simulink model "MIL4L3_SW6_V1_20220211"  (R2018b)
settings: Solver=FixedStepAuto  StartTime=0.0  StopTime=inf  FixedStep=0.001  RelTol=1e-3
PreLoadFcn:
  | A0_MILtest;
undefined symbols (not defined in the file or in its folder): Clb_ICADirect_LaneDisp_StateFive, Clb_ICADirect_LaneDisp_StateFour, Clb_ICADirect_LaneDisp_StateOne, Clb_ICADirect_LaneDisp_StateThree, Clb_ICADirect_LaneDisp_StateTwo, Clb_ICADirect_LaneDisp_StateZero, Clb_ICADirect_LaneDispSW, Clb_ICADirect_TrnLghtsCom_Switch, Clb_ICADirect_TrnLghtsCom_Value, Clb_ICADirect_TrnLghtsCrtl_Inhb, IMAP_Clb_ACU_Driver_Belt, IMAP_Clb_ACU_Driver_Belt_Over, IMAP_Clb_ACU_Passenger_Belt, IMAP_Clb_ACU_Passenger_Belt_Over, IMAP_Clb_ACU_RearLeft_Belt, IMAP_Clb_ACU_RearLeft_Belt_Over, IMAP_Clb_ACU_RearMiddle_Belt, IMAP_Clb_ACU_RearMiddle_Belt_Over, IMAP_Clb_ACU_RearRight_Belt, IMAP_Clb_ACU_RearRight_Belt_Over, IMAP_Clb_AEB_Switch, IMAP_Clb_AEB_Switch_Over, IMAP_Clb_ALC_TLC_Mode, IMAP_Clb_ALC_TLC_Mode_Over, IMAP_Clb_BCM_Battery_Voltage, IMAP_Clb_BCM_Battery_Voltage_Over, IMAP_Clb_BCM_BrakeLamp_State, IMAP_Clb_BCM_BrakeLamp_State_Over, IMAP_Clb_BCM_CHMSL_Status, IMAP_Clb_BCM_CHMSL_Status_Over, IMAP_Clb_BCM_Door_Lock_State, IMAP_Clb_BCM_Door_Lock_State_Over, IMAP_Clb_BCM_FrontWiper_State, IMAP_Clb_BCM_FrontWiper_State_Over, IMAP_Clb_BCM_FrontWiper_Switch, IMAP_Clb_BCM_FrontWiper_Switch_Over, IMAP_Clb_BCM_HazardLamp, IMAP_Clb_BCM_HazardLamp_Over, IMAP_Clb_BCM_HazardLamp_Switch, IMAP_Clb_BCM_HazardLamp_Switch_Over, IMAP_Clb_BCM_HighBeam_State, IMAP_Clb_BCM_HighBeam_State_Over, IMAP_Clb_BCM_Ignition_State, IMAP_Clb_BCM_Ignition_State_Over, IMAP_Clb_BCM_IHBC_Enabled, IMAP_Clb_BCM_IHBC_Enabled_Over, IMAP_Clb_BCM_Left_Light, IMAP_Clb_BCM_Left_Light_Over, IMAP_Clb_BCM_LeftTurn_Switch, IMAP_Clb_BCM_LeftTurn_Switch_Over, IMAP_Clb_BCM_LF_Door_State, IMAP_Clb_BCM_LF_Door_State_Over, IMAP_Clb_BCM_LowBeam_State, IMAP_Clb_BCM_LowBeam_State_Over, IMAP_Clb_BCM_LR_Door_State, IMAP_Clb_BCM_LR_Door_State_Over, IMAP_Clb_BCM_RF_Door_State, IMAP_Clb_BCM_RF_Door_State_Over, IMAP_Clb_BCM_Right_Light, IMAP_Clb_BCM_Right_Light_Over ... (+547)
libraries: CarMaker4SL x2153, simulink x292, dspstat3 x3, canmsglib x2, simulink_extras x1
(part 11 of 52)

== system MIL4L3_SW6_V1_20220211/CarMaker/VehicleControl/Function/LKA ==
  Bus Selector : BusSelector  OutputSignals=IMAPve_d_LKA_Main_Switch,IMAPve_d_LKA_Mode,IMAPve_d_LDW_Warn_Mode,IMAPve_d_APA_AutoPark_WorkSt,IMAPve_d_MP5_Work_State,IMAPve_d_EPS_LKA_State,IMAPve_g_EPS_SW_Trq,IMAPve_d_EPS_Trq_State,IMAPve_d_SAS_Clb_State,IMAPve_d_SAS_Trim_State,IMAPve_d_SWS_Failure_Status,IMAPve_d_EPS_TrqLim_State,IMAPve_g_EPS_LKA_Current,IMAPve_d_EPS_Steer_Hold_State,IMAPve_d_EPS_Driver_Override,IMAPve_d_EPS_ESA_State,IMAPve_d_EPS_SteeringAngle_Flag,IMAPve_g_EPS_SteeringAngle,IMAPve_g_SW_Angle,IMAPve_g_SW_Angle_Speed,IMAPve_g_ESC_LatAcc,IMAPve_d_ESC_LatAcc_Valid,IMAPve_g_ESC_YawRate,IMAPve_d_ESC_YawRate_Valid,IMAPve_g_ESC_UnYawRate,IMAPve_g_ESC_VehSpd,IMAPve_g_ESC_LonAcc,IMAPve_d_ESC_LonAcc_Valid,IMAPve_g_ESC_Brake_Press,IMAPve_d_ESC_VehSpd_Valid,IMAPve_d_BCM_HazardLamp,IMAPve_d_BCM_Left_Light,IMAPve_d_BCM_Right_Light,IMAPve_d_BCM_LeftTurn_Switch,IMAPve_d_BCM_RightTurn_Switch,IMAPve_d_BCM_HazardLamp_Switch,IMAPve_g_EMS_RealPedal,IMAPve_d_TCU_Actual_Gear,IMAPve_d_TCU_TCU_Available
  Bus Selector1 : BusSelector  OutputSignals=FDMMve_d_LkaFcnConf
  Bus Selector2 : BusSelector  OutputSignals=IMAPve_d_Camera_Status,IMAPve_d_Sensor_Status,IMAPve_d_Fusion_Status,IMAPve_g_L0_C0,IMAPve_g_L0_C1,IMAPve_g_L0_C2,IMAPve_g_L0_C3,IMAPve_g_L0_VR,IMAPve_d_L0_Q,IMAPve_d_L0_Type,IMAPve_g_L0_W,IMAPve_g_R0_C0,IMAPve_g_R0_C1,IMAPve_g_R0_C2,IMAPve_g_R0_C3,IMAPve_g_R0_VR,IMAPve_d_R0_Q,IMAPve_d_R0_Type,IMAPve_g_R0_W,IMAPve_g_L1_C0,IMAPve_g_L1_C1,IMAPve_g_L1_C2,IMAPve_g_L1_C3,IMAPve_g_L1_VR,IMAPve_d_L1_Q,IMAPve_d_L1_Type,IMAPve_g_L1_W,IMAPve_g_R1_C0,IMAPve_g_R1_C1,IMAPve_g_R1_C2,IMAPve_g_R1_C3,IMAPve_g_R1_VR,IMAPve_d_R1_Q,IMAPve_d_R1_Type,IMAPve_g_R1_W
  BusCreator : BusCreator  Inputs=13
  EPS_State_Mashine : Subsystem
  LKAS1 : Subsystem  TreatAsAtomicUnit=on
  Memory : Memory
  tag scope: EPS_LKA_State_lka=global, LKA_output=global
  wires:
  BusCreator/1 -> [LKA_output]
  [IMAP_Output] -> Bus Selector/1, Bus Selector2/1
  Bus Selector1/1 -> LKAS1/1(FDMMve_d_LkaFcnConf)  "<FDMMve_d_LkaFcnConf>"
  [FDMM_output] -> Bus Selector1/1
  Memory/1 -> [EPS_LKA_State_lka]
  EPS_State_Mashine/1(EPS_Ctr_State) -> Memory/1
  Bus Selector/2 -> LKAS1/3(IMAPve_d_LKA_Mode)  "<IMAPve_d_LKA_Mode>"
  Bus Selector/3 -> LKAS1/4(IMAPve_d_LDW_Warn_Mode)  "<IMAPve_d_LDW_Warn_Mode>"
  Bus Selector/1 -> LKAS1/2(IMAPve_d_LKA_Main_Switch)  "<IMAPve_d_LKA_Main_Switch>"
  Bus Selector/4 -> LKAS1/5(IMAPve_d_APA_AutoPark_WorkSt)  "<IMAPve_d_APA_AutoPark_WorkSt>"
  Bus Selector/5 -> LKAS1/6(IMAPve_d_MP5_Work_State)  "<IMAPve_d_MP5_Work_State>"
  Bus Selector/6 -> LKAS1/7(IMAPve_d_EPS_LKA_State)  "<IMAPve_d_EPS_LKA_State>"
  Bus Selector/7 -> LKAS1/8(IMAPve_g_EPS_SW_Trq)  "<IMAPve_g_EPS_SW_Trq>"
  Bus Selector/8 -> LKAS1/9(IMAPve_d_EPS_Trq_State)  "<IMAPve_d_EPS_Trq_State>"
  Bus Selector/9 -> LKAS1/10(IMAPve_d_SAS_Clb_State)  "<IMAPve_d_SAS_Clb_State>"
  Bus Selector/10 -> LKAS1/11(IMAPve_d_SAS_Trim_State)  "<IMAPve_d_SAS_Trim_State>"
  Bus Selector/11 -> LKAS1/12(IMAPve_d_SWS_Failure_Status)  "<IMAPve_d_SWS_Failure_Status>"
  Bus Selector/12 -> LKAS1/13(IMAPve_d_EPS_TrqLim_State)  "<IMAPve_d_EPS_TrqLim_State>"
  Bus Selector/13 -> LKAS1/14(IMAPve_g_EPS_LKA_Current)  "<IMAPve_g_EPS_LKA_Current>"
  Bus Selector/14 -> LKAS1/15(IMAPve_d_EPS_Steer_Hold_State)  "<IMAPve_d_EPS_Steer_Hold_State>"
  Bus Selector/15 -> LKAS1/16(IMAPve_d_EPS_Driver_Override)  "<IMAPve_d_EPS_Driver_Override>"
  Bus Selector/16 -> LKAS1/17(IMAPve_d_EPS_ESA_State)  "<IMAPve_d_EPS_ESA_State>"
  Bus Selector/17 -> LKAS1/18(IMAPve_d_EPS_SteeringAngle_Flag)  "<IMAPve_d_EPS_SteeringAngle_Flag>"
  Bus Selector/18 -> LKAS1/19(IMAPve_g_EPS_SteeringAngle)  "<IMAPve_g_EPS_SteeringAngle>"
  Bus Selector/19 -> LKAS1/20(IMAPve_g_SW_Angle)  "<IMAPve_g_SW_Angle>"
  Bus Selector/20 -> LKAS1/21(IMAPve_g_SW_Angle_Speed)  "<IMAPve_g_SW_Angle_Speed>"
  Bus Selector/21 -> LKAS1/22(IMAPve_g_ESC_LatAcc)  "<IMAPve_g_ESC_LatAcc>"
  Bus Selector/22 -> LKAS1/23(IMAPve_d_ESC_LatAcc_Valid)  "<IMAPve_d_ESC_LatAcc_Valid>"
  Bus Selector/23 -> LKAS1/24(IMAPve_g_ESC_YawRate)  "<IMAPve_g_ESC_YawRate>"
  Bus Selector/24 -> LKAS1/25(IMAPve_d_ESC_YawRate_Valid)  "<IMAPve_d_ESC_YawRate_Valid>"
  Bus Selector/25 -> LKAS1/26(IMAPve_g_ESC_UnYawRate)  "<IMAPve_g_ESC_UnYawRate>"
  Bus Selector/26 -> LKAS1/27(IMAPve_g_ESC_VehSpd)  "<IMAPve_g_ESC_VehSpd>"
  Bus Selector/27 -> LKAS1/28(IMAPve_g_ESC_LonAcc)  "<IMAPve_g_ESC_LonAcc>"
  Bus Selector/28 -> LKAS1/29(IMAPve_d_ESC_LonAcc_Valid)  "<IMAPve_d_ESC_LonAcc_Valid>"
  Bus Selector/29 -> LKAS1/30(IMAPve_g_ESC_Brake_Press)  "<IMAPve_g_ESC_Brake_Press>"
  Bus Selector/30 -> LKAS1/31(IMAPve_d_ESC_VehSpd_Valid)  "<IMAPve_d_ESC_VehSpd_Valid>"
  Bus Selector/31 -> LKAS1/32(IMAPve_d_BCM_HazardLamp)  "<IMAPve_d_BCM_HazardLamp>"
  Bus Selector/32 -> LKAS1/33(IMAPve_d_BCM_Left_Light)  "<IMAPve_d_BCM_Left_Light>"
  Bus Selector/33 -> LKAS1/34(IMAPve_d_BCM_Right_Light)  "<IMAPve_d_BCM_Right_Light>"
  Bus Selector/34 -> LKAS1/35(IMAPve_d_BCM_LeftTurn_Switch)  "<IMAPve_d_BCM_LeftTurn_Switch>"
  Bus Selector/35 -> LKAS1/36(IMAPve_d_BCM_RightTurn_Switch)  "<IMAPve_d_BCM_RightTurn_Switch>"
  Bus Selector/36 -> LKAS1/37(IMAPve_d_BCM_HazardLamp_Switch)  "<IMAPve_d_BCM_HazardLamp_Switch>"
  Bus Selector/37 -> LKAS1/38(IMAPve_g_EMS_RealPedal)  "<IMAPve_g_EMS_RealPedal>"
  Bus Selector/38 -> LKAS1/39(IMAPve_d_TCU_Actual_Gear)  "<IMAPve_d_TCU_Actual_Gear>"
  Bus Selector/39 -> LKAS1/40(IMAPve_d_TCU_TCU_Available)  "<IMAPve_d_TCU_TCU_Available>"
  ? -> LKAS1/41(ADIAve_g_ASWFaultStatus)
  ? -> LKAS1/42(ADIAve_g_BSWFaultStatus)
  ? -> LKAS1/43(ADIAve_d_FuncFaultStatus)
  Bus Selector2/1 -> LKAS1/44(IMAPve_d_Camera_Status)  "<IMAPve_d_Camera_Status>"
  Bus Selector2/2 -> LKAS1/45(IMAPve_d_Sensor_Status)  "<IMAPve_d_Sensor_Status>"
  Bus Selector2/3 -> LKAS1/46(IMAPve_d_Fusion_Status)  "<IMAPve_d_Fusion_Status>"
  Bus Selector2/4 -> LKAS1/47(IMAPve_g_L0_C0)  "<IMAPve_g_L0_C0>"
  Bus Selector2/5 -> LKAS1/48(IMAPve_g_L0_C1)  "<IMAPve_g_L0_C1>"
  Bus Selector2/6 -> LKAS1/49(IMAPve_g_L0_C2)  "<IMAPve_g_L0_C2>"
  Bus Selector2/7 -> LKAS1/50(IMAPve_g_L0_C3)  "<IMAPve_g_L0_C3>"
  Bus Selector2/8 -> LKAS1/51(IMAPve_g_L0_VR)  "<IMAPve_g_L0_VR>"
  Bus Selector2/9 -> LKAS1/52(IMAPve_d_L0_Q)  "<IMAPve_d_L0_Q>"
  Bus Selector2/10 -> LKAS1/53(IMAPve_d_L0_Type)  "<IMAPve_d_L0_Type>"
  Bus Selector2/11 -> LKAS1/54(IMAPve_g_L0_W)  "<IMAPve_g_L0_W>"
  Bus Selector2/12 -> LKAS1/55(IMAPve_g_R0_C0)  "<IMAPve_g_R0_C0>"
  Bus Selector2/13 -> LKAS1/56(IMAPve_g_R0_C1)  "<IMAPve_g_R0_C1>"
  Bus Selector2/14 -> LKAS1/57(IMAPve_g_R0_C2)  "<IMAPve_g_R0_C2>"
  Bus Selector2/15 -> LKAS1/58(IMAPve_g_R0_C3)  "<IMAPve_g_R0_C3>"
  Bus Selector2/16 -> LKAS1/59(IMAPve_g_R0_VR)  "<IMAPve_g_R0_VR>"
  Bus Selector2/17 -> LKAS1/60(IMAPve_d_R0_Q)  "<IMAPve_d_R0_Q>"
  Bus Selector2/18 -> LKAS1/61(IMAPve_d_R0_Type)  "<IMAPve_d_R0_Type>"
  Bus Selector2/19 -> LKAS1/62(IMAPve_g_R0_W)  "<IMAPve_g_R0_W>"
  Bus Selector2/20 -> LKAS1/63(IMAPve_g_L1_C0)  "<IMAPve_g_L1_C0>"
  Bus Selector2/21 -> LKAS1/64(IMAPve_g_L1_C1)  "<IMAPve_g_L1_C1>"
  Bus Selector2/22 -> LKAS1/65(IMAPve_g_L1_C2)  "<IMAPve_g_L1_C2>"
  Bus Selector2/23 -> LKAS1/66(IMAPve_g_L1_C3)  "<IMAPve_g_L1_C3>"
  Bus Selector2/24 -> LKAS1/67(IMAPve_g_L1_VR)  "<IMAPve_g_L1_VR>"
  Bus Selector2/25 -> LKAS1/68(IMAPve_d_L1_Q)  "<IMAPve_d_L1_Q>"
  Bus Selector2/26 -> LKAS1/69(IMAPve_d_L1_Type)  "<IMAPve_d_L1_Type>"
  Bus Selector2/27 -> LKAS1/70(IMAPve_g_L1_W)  "<IMAPve_g_L1_W>"
  Bus Selector2/28 -> LKAS1/71(IMAPve_g_R1_C0)  "<IMAPve_g_R1_C0>"
  Bus Selector2/29 -> LKAS1/72(IMAPve_g_R1_C1)  "<IMAPve_g_R1_C1>"
  Bus Selector2/30 -> LKAS1/73(IMAPve_g_R1_C2)  "<IMAPve_g_R1_C2>"
  Bus Selector2/31 -> LKAS1/74(IMAPve_g_R1_C3)  "<IMAPve_g_R1_C3>"
  Bus Selector2/32 -> LKAS1/75(IMAPve_g_R1_VR)  "<IMAPve_g_R1_VR>"
  Bus Selector2/33 -> LKAS1/76(IMAPve_d_R1_Q)  "<IMAPve_d_R1_Q>"
  Bus Selector2/34 -> LKAS1/77(IMAPve_d_R1_Type)  "<IMAPve_d_R1_Type>"
  Bus Selector2/35 -> LKAS1/78(IMAPve_g_R1_W)  "<IMAPve_g_R1_W>"
  LKAS1/6(LKASve_y_LKA_Action_Indication) -> BusCreator/6  "LKASve_y_LKA_Action_Indication"
  LKAS1/7(LKASve_y_HMI_Popup_Status) -> BusCreator/7  "LKASve_y_HMI_Popup_Status"
  LKAS1/5(LKASve_y_Hands_Off_Warning) -> BusCreator/5  "LKASve_y_Hands_Off_Warning"
  LKAS1/8(LKASve_y_LKATorqueReq) -> BusCreator/8  "LKASve_y_LKATorqueReq"
  LKAS1/4(LKASve_y_LDW_Flag) -> BusCreator/4  "LKASve_y_LDW_Flag"
  LKAS1/9(LKASve_g_LKATorqueReq_Value) -> BusCreator/9  "LKASve_g_LKATorqueReq_Value"
  LKAS1/3(LKASve_y_LKA_Status_Display) -> BusCreator/3  "LKASve_y_LKA_Status_Display"
  LKAS1/10(LKASve_y_EPS_State_Control) -> BusCreator/10, EPS_State_Mashine/1(LKA_State2EPS)  "LKASve_y_EPS_State_Control"
  LKAS1/2(LKASve_y_LDW_Status_Display) -> BusCreator/2  "LKASve_y_LDW_Status_Display"
  LKAS1/11(LKASve_g_LKA_SWA_Control) -> BusCreator/11  "LKASve_g_LKA_SWA_Control"
  LKAS1/1(LKASve_y_Vehicle_Lane_Display) -> BusCreator/1  "LKASve_y_Vehicle_Lane_Display"
  LKAS1/12(LKASve_g_EPS_Factor_Control) -> BusCreator/12  "LKASve_g_EPS_Factor_Control"
  LKAS1/13(LKASve_y_EPS_LKA_Control) -> BusCreator/13  "LKASve_y_EPS_LKA_Control"

== system MIL4L3_SW6_V1_20220211/CarMaker/VehicleControl/FunctionDataLog/ACC ==
  Bus Selector12 : BusSelector  OutputSignals=IMAPve_d_ESC_FLW_Direction,IMAPve_d_ESC_FRW_Direction,IMAPve_d_ESC_TCS_ErrorStatus,IMAPve_d_ESC_RLW_Direction,IMAPve_d_ESC_RRW_Direction,IMAPve_d_ESC_EPB_ErrorStatus,IMAPve_d_EPS_SteeringAngle_Flag,IMAPve_g_EPS_SteeringAngle,IMAPve_d_EPS_Driver_Override,IMAPve_d_EPS_Driver_Active_ESA,IMAPve_d_EPS_ESA_State,IMAPve_d_ACU_RearLeft_Belt,IMAPve_d_ACU_RearMiddle_Belt,IMAPve_d_ACU_RearRight_Belt,IMAPve_d_EMS_PowertrainCtl_State,IMAPve_d_TCU_TCU_Available,IMAPve_d_BCM_LeftTurn_Switch,IMAPve_d_BCM_RightTurn_Switch,IMAPve_d_BCM_FrontWiper_Switch,IMAPve_d_BCM_IHBC_Enabled,IMAPve_d_MP5_Work_State,IMAPve_d_MP5_APA_ModeSelect,IMAPve_d_MP5_LanguageSet,IMAPve_d_MP5_UPA_Switch,IMAPve_d_MP5_FLK_Activation,IMAPve_d_MP5_AutoPilot_Switch,IMAPve_d_MP5_DMS_MessageType,IMAPve_d_MP5_DMS_SystemEnable,IMAPve_d_MP5_DMS_DelUserNum,IMAPve_d_MP5_DMS_Sensity,IMAPve_d_MP5_DMS_EyeFatigue,IMAPve_d_MP5_DMS_LongtimeDrive,IMAPve_d_MP5_DMS_SideView,IMAPve_d_MP5_DMS_UsingPhone,IMAPve_d_MP5_DMS_Smoking,IMAPve_d_MP5_DMS_DrinkWater,IMAPve_d_MP5_DMS_UserAccount
  Bus Selector : BusSelector  OutputSignals=IMAPve_d_ISA_Switch,IMAPve_d_TSR_Switch,IMAPve_d_ISA_ISLC_Mode,IMAPve_d_Speed_Limit,IMAPve_d_ALC_TLC_Mode,IMAPve_d_PEPS_RKE_Command,IMAPve_d_DOW_Switch,IMAPve_d_LF_Switch,IMAPve_d_ICA_Config,IMAPve_d_ALC_Sensitivity
  Bus Selector1 : BusSelector  OutputSignals=IMAPve_d_Sensor_Status,IMAPve_d_LF_Radar_Status,IMAPve_d_RF_Radar_Status,IMAPve_d_LR_Radar_Status,IMAPve_d_RR_Radar_Status,IMAPve_d_Fusion_Status,IMAPve_g_Fusion_Time_Stamp,IMAPve_d_obj_Num,IMAPva_d_obj_id,IMAPva_g_obj_pos_x,IMAPva_g_obj_pos_y,IMAPva_g_obj_vel_x,IMAPva_g_obj_vel_y,IMAPva_g_obj_acc_x,IMAPva_g_obj_acc_y,IMAPva_g_obj_pos_var_x,IMAPva_g_obj_pos_var_y,IMAPva_g_obj_pos_var_xy,IMAPva_g_obj_width,IMAPva_g_obj_length,IMAPva_d_obj_class,IMAPva_d_obj_lane,IMAPva_d_obj_status,IMAPva_d_obj_age,IMAPva_d_obj_TurnLight,IMAPva_d_obj_BrakeLight,IMAPva_d_obj_MotionStatus,IMAPve_d_Lane_Valid,IMAPve_d_Road_Type,IMAPve_d_ConsArea,IMAPve_g_L0_C0,IMAPve_g_L0_C1,IMAPve_g_L0_C2,IMAPve_g_L0_C3,IMAPve_g_L0_VR,IMAPve_d_L0_Q,IMAPve_d_L0_Type,IMAPve_g_L0_Confidence,IMAPve_g_L0_W,IMAPve_g_L0_TLC,IMAPve_d_L0_LC,IMAPve_g_R0_C0,IMAPve_g_R0_C1,IMAPve_g_R0_C2,IMAPve_g_R0_C3,IMAPve_g_R0_VR,IMAPve_d_R0_Q,IMAPve_d_R0_Type,IMAPve_g_R0_Confidence,IMAPve_g_R0_W,IMAPve_g_R0_TLC,IMAPve_d_R0_LC,IMAPve_g_L1_C0,IMAPve_g_L1_C1,IMAPve_g_L1_C2,IMAPve_g_L1_C3,IMAPve_g_L1_VR,IMAPve_d_L1_Q,IMAPve_d_L1_Type,IMAPve_g_L1_Confidence,IMAPve_g_L1_W,IMAPve_g_L1_TLC,IMAPve_d_L1_LC,IMAPve_g_R1_C0,IMAPve_g_R1_C1,IMAPve_g_R1_C2,IMAPve_g_R1_C3,IMAPve_g_R1_VR,IMAPve_d_R1_Q,IMAPve_d_R1_Type,IMAPve_g_R1_Confidence,IMAPve_g_R1_W,IMAPve_g_R1_TLC,IMAPve_d_R1_LC,IMAPve_g_L0_C0_Back,IMAPve_g_L0_C1_Back,IMAPve_g_L0_C2_Back,IMAPve_g_L0_C3_Back,IMAPve_g_L0_Range_Back,IMAPve_g_L0_C0_FR_Pred,IMAPve_g_L0_C1_FR_Pred,IMAPve_g_L0_C2_FR_Pred,IMAPve_g_L0_Range_FR_Pred,IMAPve_g_R0_C0_Back,IMAPve_g_R0_C1_Back,IMAPve_g_R0_C2_Back,IMAPve_g_R0_C3_Back,IMAPve_g_R0_Range_Back,IMAPve_g_R0_C0_FR_Pred,IMAPve_g_R0_C1_FR_Pred,IMAPve_g_R0_C2_FR_Pred,IMAPve_g_R0_Range_FR_Pred,IMAPve_g_L1_C0_Back,IMAPve_g_L1_C1_Back,IMAPve_g_L1_C2_Back,IMAPve_g_L1_C3_Back,IMAPve_g_L1_Range_Back,IMAPve_g_L1_C0_FR_Pred,IMAPve_g_L1_C1_FR_Pred,IMAPve_g_L1_C2_FR_Pred,IMAPve_g_L1_Range_FR_Pred,IMAPve_g_R1_C0_Back,IMAPve_g_R1_C1_Back,IMAPve_g_R1_C2_Back,IMAPve_g_R1_C3_Back,IMAPve_g_R1_Range_Back,IMAPve_g_R1_C0_FR_Pred,IMAPve_g_R1_C1_FR_Pred,IMAPve_g_R1_C2_FR_Pred,IMAPve_g_R1_Range_FR_Pred,IMAPve_d_Sign_ISA_Value,IMAPve_d_TSR_Sign_Type,IMAPve_d_Camera_Signal_Fault,IMAPve_d_Radar_Status,IMAPve_d_Camera_Status
  Bus Selector10 : BusSelector  OutputSignals=IMAPve_d_ORI_CIPV_ID,IMAPve_d_ORI_Obj_Num,IMAPva_g_ORI_Probability,IMAPva_d_ORI_Obj_Class,IMAPva_d_ORI_Obj_Motion,IMAPva_g_ORI_Obj_RelVel,IMAPva_g_ORI_Obj_LongDis,IMAPva_d_ORI_Obj_Lane,IMAPva_g_ORI_Obj_LAngle,IMAPva_g_ORI_Obj_RAngle,IMAPva_g_ORI_Obj_Width,IMAPva_d_ORI_Obj_ID
  Bus Selector11 : BusSelector  OutputSignals=IMAPve_d_ORI_Lane_Valid,IMAPve_d_ORI_Lane_ConsArea,IMAPve_d_ORI_Lane_RoadType,IMAPve_g_ORI_L0_C3,IMAPve_g_ORI_L0_C2,IMAPve_g_ORI_L0_C1,IMAPve_g_ORI_L0_C0,IMAPve_d_ORI_L0_Q,IMAPve_d_ORI_L0_Type,IMAPve_g_ORI_L0_VR,IMAPve_g_ORI_L0_TLC,IMAPve_g_ORI_L0_W,IMAPve_d_ORI_L0_LC,IMAPve_g_ORI_L1_C3,IMAPve_g_ORI_L1_C2,IMAPve_g_ORI_L1_C1,IMAPve_g_ORI_L1_C0,IMAPve_d_ORI_L1_Q,IMAPve_d_ORI_L1_Type,IMAPve_g_ORI_L1_VR,IMAPve_g_ORI_L1_TLC,IMAPve_g_ORI_L1_W,IMAPve_d_ORI_L1_LC,IMAPve_g_ORI_R0_C3,IMAPve_g_ORI_R0_C2,IMAPve_g_ORI_R0_C1,IMAPve_g_ORI_R0_C0,IMAPve_d_ORI_R0_Q,IMAPve_d_ORI_R0_LT,IMAPve_g_ORI_R0_VR,IMAPve_g_ORI_R0_TLC,IMAPve_g_ORI_R0_W,IMAPve_d_ORI_R0_LC,IMAPve_g_ORI_R1_C3,IMAPve_g_ORI_R1_C2,IMAPve_g_ORI_R1_C1,IMAPve_g_ORI_R1_C0,IMAPve_d_ORI_R1_Q,IMAPve_d_ORI_R1_LT,IMAPve_g_ORI_R1_VR,IMAPve_g_ORI_R1_TLC,IMAPve_g_ORI_R1_W,IMAPve_d_ORI_R1_LC
  Bus Selector2 : BusSelector  OutputSignals=ICASva_g_ExceptAcc,ICASve_d_ExceptAccValidNum,ICASve_d_ExceptAccValid,ICASva_d_TrajectoryPlanState,ICASve_g_ExpLonAcc,ICASve_d_SignalTStamp
  Bus Selector3 : BusSelector  OutputSignals=IMAPve_d_EPS_LKA_State,IMAPve_g_EPS_SW_Trq,IMAPve_d_EPS_Error_State,IMAPve_d_EPS_Trq_State,IMAPve_d_SAS_Clb_State,IMAPve_d_SAS_Trim_State,IMAPve_d_EPS_TrqLim_State,IMAPve_g_EPS_LKA_Current
  Bus Selector4 : BusSelector  OutputSignals=IMAPve_g_ESC_LatAcc,IMAPve_d_ESC_LatAcc_Valid,IMAPve_g_ESC_YawRate,IMAPve_d_ESC_YawRate_Valid,IMAPve_g_ESC_UnYawRate,IMAPve_g_ESC_VehSpd,IMAPve_g_ESC_LonAcc,IMAPve_d_ESC_LonAcc_Valid,IMAPve_g_ESC_Brake_Press,IMAPve_g_ESC_Static_Slope,IMAPve_g_ESC_DySlope_Accuracy,IMAPve_g_ESC_DySlope
  Bus Selector5 : BusSelector  OutputSignals=IMAPve_g_SW_Angle,IMAPve_g_SW_Angle_Speed
  Bus Selector6 : BusSelector  OutputSignals=IMAPve_d_BCM_HazardLamp,IMAPve_d_BCM_Left_Light,IMAPve_d_BCM_Right_Light,IMAPve_d_ESC_BrakeLamp_Req,IMAPve_d_BCM_Opening_State,IMAPve_d_BCM_Trunk_State,IMAPve_d_BCM_LF_Door_State,IMAPve_d_BCM_RF_Door_State,IMAPve_d_BCM_RR_Door_State,IMAPve_d_BCM_LR_Door_State
  Bus Selector7 : BusSelector  OutputSignals=IMAPve_d_SCC_Left_SwitchSig,IMAPve_d_SCC_Right_SwitchSig,IMAPve_d_PEPS_Door_Lock_Req,IMAPve_d_BCM_Door_Lock_State
  Bus Selector8 : BusSelector  OutputSignals=IMAPve_d_EMS_ACC_Status,IMAPve_g_EMS_Pot_WhlT_Max,IMAPve_g_EMS_Pot_WhlT_Min,IMAPve_g_EMS_RealPedal,IMAPve_g_EMS_MaxTWhl,IMAPve_g_EMS_MaxTWhl_Offset,IMAPve_g_EMS_MinTWhl,IMAPve_g_EMS_MinTWhl_Offset,IMAPve_g_EMS_Actual_FlwT,IMAPve_g_EMS_Actual_IndT,IMAPve_g_EMS_Realize_TWhl,IMAPve_g_EMS_ACC_VirtualPedal,IMAPve_d_EMS_AccPedal_Fault,IMAPve_g_EMS_Driver_Torque,IMAPve_d_ESC_Brake_Effort,IMAPve_g_EMS_Engine_Speed,IMAPve_d_ESC_Veh_Standstill,IMAPve_d_TCU_Actual_Gear,IMAPve_d_TCU_Target_Gear,IMAPve_d_TCU_PRND_State
  Bus Selector9 : BusSelector  OutputSignals=IMAPve_d_BCM_Ignition_State,IMAPve_d_ACU_Driver_Belt,IMAPve_d_SWS_Fault_Code,IMAPve_d_SWS_Failure_Status,IMAPve_d_ESC_OFF,IMAPve_d_ESC_AlarmSig,IMAPve_d_Speed_Limit_Switch,IMAPve_d_ESC_ESC_Active,IMAPve_d_ESC_MSR_Active,IMAPve_d_ESC_TCS_Active,IMAPve_d_ESC_VehSpd_Valid,IMAPve_d_Brake_Pedal_Fault,IMAPve_d_ESC_ABS_Active,IMAPve_d_ESC_ABS_Valid,IMAPve_d_ESC_ABS_AlarmSig,IMAPve_d_ESC_FL_WheelPulVal,IMAPve_d_ESC_FR_WheelPulVal,IMAPve_d_ESC_RL_WheelPulVal,IMAPve_d_ESC_RR_WheelPulVal,IMAPve_g_ESC_FL_WhlSpd,IMAPve_d_ESC_FL_WhlSpd_Fault,IMAPve_g_ESC_FR_WhlSpd,IMAPve_d_ESC_FR_WhlSpd_Fault,IMAPve_g_ESC_RL_WhlSpd,IMAPve_d_ESC_RL_WhlSpd_Fault,IMAPve_g_ESC_RR_WhlSpd,IMAPve_d_ESC_RR_WhlSpd_Fault,IMAPve_d_ESC_FL_Wheel_Pulse,IMAPve_d_ESC_FR_Wheel_Pulse,IMAPve_d_ESC_RL_Wheel_Pulse,IMAPve_d_ESC_RR_Wheel_Pulse,IMAPve_d_TCU_AT_Failure,IMAPve_d_TCU_Shift_Valid,IMAPve_d_TCU_DCT_Clutch_State,IMAPve_d_TCU_Gear_Engage,IMAPve_d_TCU_Select_ATMode,IMAPve_d_EMS_Engine_Status,IMAPve_d_EMS_Gearbox_CtlAvail,IMAPve_d_ESC_Brake_Failsafe,IMAPve_d_ESC_AEB_Status,IMAPve_d_ESC_AEB_Available,IMAPve_d_ESC_AEB_Active,IMAPve_d_ESC_ACC_Status,IMAPve_d_ESC_ACC_Available,IMAPve_d_ESC_ACC_Active,IMAPve_d_EMS_ACC_Effective,IMAPve_d_BCM_FrontWiper_State,IMAPve_d_BCM_CHMSL_Status,IMAPve_d_BCM_BrakeLamp_State,IMAPve_d_GW_Brake_Only_Req,IMAPve_d_ACU_Passenger_Belt,IMAPve_d_EMS_ACC_CtlAvail,IMAPve_d_EMS_ACC_Inhibited,IMAPve_d_EMS_Brake_Pedal,IMAPve_d_BCM_LowBeam_State,IMAPve_d_BCM_HighBeam_State,IMAPve_d_EPB_Status,IMAPve_d_EPB_Display_Req,IMAPve_d_EPB_Warn_Req,IMAPve_d_EPB_Switch_State,IMAPve_d_EPB_Switch_Valid,IMAPve_d_ESC_Drive_Direction,IMAPve_d_ESC_Hold_State,IMAPve_d_EPS_Steer_Hold_State,IMAPve_d_EPS_Warning_State,IMAPve_g_EPS_PowerCon,IMAPve_d_ESC_EBD_AlarmSig,IMAPve_d_ESC_AVH_Status,IMAPve_d_Radar_Detective_Req,IMAPve_g_BCM_Battery_Voltage,IMAPve_d_TBOX_LocalTimeY,IMAPve_d_TBOX_LocalTimeM,IMAPve_d_TBOX_LocalTimeD,IMAPve_d_TBOX_LocalTimeH,IMAPve_d_TBOX_LocalTimeMin,IMAPve_d_TBOX_LocalTimeS,IMAPve_d_TBOX_LocalTime_Valid,IMAPve_d_TPMS_Warn_Indicate,IMAPve_d_Radar_State,IMAPve_d_ACC_Desired_Headway,IMAPve_d_Time_System_Clock,IMAPve_d_Signal_Time_Stamp,IMAPve_g_GW_IC_Odometer,IMAPve_g_FAPA_State,IMAPve_d_Outside_Temp
  BusCreator : BusCreator  Inputs=373
  Clock : Clock
  Data Type Conversion : DataTypeConversion
  Ground{1..4} (4 alike) : Ground
  Terminator : Terminator
  To Workspace : ToWorkspace  VariableName=ACCDataLog  SaveFormat=Timeseries  SampleTime=-1
  wires:
  [AEBSve_d_MDDdecRequest] -> BusCreator/152
  [IMAPve_g_ESC_BrkWhlCylinder_Pressure] -> BusCreator/373  "IMAPve_g_ESC_BrkWhlCylinder_Pressure"
  [IMAPve_d_APA_AutoPark_WorkSt] -> BusCreator/372  "IMAPve_d_APA_AutoPark_WorkSt"
  Bus Selector12/37 -> BusCreator/371  "<IMAPve_d_MP5_DMS_UserAccount>"
  Bus Selector12/36 -> BusCreator/370  "<IMAPve_d_MP5_DMS_DrinkWater>"
  Bus Selector12/35 -> BusCreator/369  "<IMAPve_d_MP5_DMS_Smoking>"
  Bus Selector12/34 -> BusCreator/368  "<IMAPve_d_MP5_DMS_UsingPhone>"
  Bus Selector12/33 -> BusCreator/367  "<IMAPve_d_MP5_DMS_SideView>"
  Bus Selector12/32 -> BusCreator/366  "<IMAPve_d_MP5_DMS_LongtimeDrive>"
  Bus Selector12/31 -> BusCreator/365  "<IMAPve_d_MP5_DMS_EyeFatigue>"
  Bus Selector12/30 -> BusCreator/364  "<IMAPve_d_MP5_DMS_Sensity>"
  Bus Selector12/29 -> BusCreator/363  "<IMAPve_d_MP5_DMS_DelUserNum>"
  Bus Selector12/28 -> BusCreator/362  "<IMAPve_d_MP5_DMS_SystemEnable>"
  Bus Selector12/27 -> BusCreator/361  "<IMAPve_d_MP5_DMS_MessageType>"
  Bus Selector12/26 -> BusCreator/360  "<IMAPve_d_MP5_AutoPilot_Switch>"
  Bus Selector12/25 -> BusCreator/359  "<IMAPve_d_MP5_FLK_Activation>"
  Bus Selector12/24 -> BusCreator/358  "<IMAPve_d_MP5_UPA_Switch>"
  Bus Selector12/23 -> BusCreator/357  "<IMAPve_d_MP5_LanguageSet>"
  Bus Selector12/22 -> BusCreator/356  "<IMAPve_d_MP5_APA_ModeSelect>"
  Bus Selector12/21 -> BusCreator/355  "<IMAPve_d_MP5_Work_State>"
  Bus Selector12/20 -> BusCreator/354  "<IMAPve_d_BCM_IHBC_Enabled>"
  Bus Selector12/19 -> BusCreator/353  "<IMAPve_d_BCM_FrontWiper_Switch>"
  Bus Selector12/18 -> BusCreator/352  "<IMAPve_d_BCM_RightTurn_Switch>"
  Bus Selector12/17 -> BusCreator/351  "<IMAPve_d_BCM_LeftTurn_Switch>"
  Bus Selector12/16 -> BusCreator/350  "<IMAPve_d_TCU_TCU_Available>"
  Bus Selector12/15 -> BusCreator/349  "<IMAPve_d_EMS_PowertrainCtl_State>"
  Bus Selector12/14 -> BusCreator/348  "<IMAPve_d_ACU_RearRight_Belt>"
  Bus Selector12/13 -> BusCreator/347  "<IMAPve_d_ACU_RearMiddle_Belt>"
  Bus Selector12/12 -> BusCreator/346  "<IMAPve_d_ACU_RearLeft_Belt>"
  Bus Selector12/11 -> BusCreator/345  "<IMAPve_d_EPS_ESA_State>"
  Bus Selector12/10 -> BusCreator/344  "<IMAPve_d_EPS_Driver_Active_ESA>"
  Bus Selector12/9 -> BusCreator/343  "<IMAPve_d_EPS_Driver_Override>"
  Bus Selector12/8 -> BusCreator/342  "<IMAPve_g_EPS_SteeringAngle>"
  Bus Selector12/7 -> BusCreator/341  "<IMAPve_d_EPS_SteeringAngle_Flag>"
  Bus Selector12/6 -> BusCreator/340  "<IMAPve_d_ESC_EPB_ErrorStatus>"
  Bus Selector12/5 -> BusCreator/339  "<IMAPve_d_ESC_RRW_Direction>"
  Bus Selector12/4 -> BusCreator/338  "<IMAPve_d_ESC_RLW_Direction>"
  Bus Selector12/3 -> BusCreator/337  "<IMAPve_d_ESC_TCS_ErrorStatus>"
  Bus Selector12/2 -> BusCreator/336  "<IMAPve_d_ESC_FRW_Direction>"
  Bus Selector12/1 -> BusCreator/335  "<IMAPve_d_ESC_FLW_Direction>"
  [busNew] -> Bus Selector12/1
  Data Type Conversion/1 -> BusCreator/149
  Bus Selector2/2 -> BusCreator/160  "<ICASve_d_ExceptAccValidNum>"
  Bus Selector2/3 -> BusCreator/161  "<ICASve_d_ExceptAccValid>"
  Bus Selector2/4 -> BusCreator/162  "<ICASva_d_TrajectoryPlanState>"
  Bus Selector2/5 -> BusCreator/163  "<ICASve_g_ExpLonAcc>"
  Bus Selector2/6 -> BusCreator/164  "<ICASve_d_SignalTStamp>"
  Bus Selector2/1 -> BusCreator/159  "<ICASva_g_ExceptAcc>"
  Bus Selector1/115 -> BusCreator/334  "<IMAPve_d_Camera_Status>"
  Bus Selector1/114 -> BusCreator/333  "<IMAPve_d_Radar_Status>"
  Bus Selector1/113 -> BusCreator/332  "<IMAPve_d_Camera_Signal_Fault>"
  Bus Selector1/112 -> BusCreator/331  "<IMAPve_d_TSR_Sign_Type>"
  Bus Selector1/111 -> BusCreator/330  "<IMAPve_d_Sign_ISA_Value>"
  Bus Selector1/110 -> BusCreator/329  "<IMAPve_g_R1_Range_FR_Pred>"
  Bus Selector1/109 -> BusCreator/328  "<IMAPve_g_R1_C2_FR_Pred>"
  Bus Selector1/108 -> BusCreator/327  "<IMAPve_g_R1_C1_FR_Pred>"
  Bus Selector1/107 -> BusCreator/326  "<IMAPve_g_R1_C0_FR_Pred>"
  Bus Selector1/106 -> BusCreator/325  "<IMAPve_g_R1_Range_Back>"
  Bus Selector1/105 -> BusCreator/324  "<IMAPve_g_R1_C3_Back>"
  Bus Selector1/104 -> BusCreator/323  "<IMAPve_g_R1_C2_Back>"
  Bus Selector1/103 -> BusCreator/322  "<IMAPve_g_R1_C1_Back>"
  Bus Selector1/102 -> BusCreator/321  "<IMAPve_g_R1_C0_Back>"
  Bus Selector1/101 -> BusCreator/320  "<IMAPve_g_L1_Range_FR_Pred>"
  Bus Selector1/100 -> BusCreator/319  "<IMAPve_g_L1_C2_FR_Pred>"
  Bus Selector1/99 -> BusCreator/318  "<IMAPve_g_L1_C1_FR_Pred>"
  Bus Selector1/98 -> BusCreator/317  "<IMAPve_g_L1_C0_FR_Pred>"
  Bus Selector1/97 -> BusCreator/316  "<IMAPve_g_L1_Range_Back>"
  Bus Selector1/96 -> BusCreator/315  "<IMAPve_g_L1_C3_Back>"
  Bus Selector1/95 -> BusCreator/314  "<IMAPve_g_L1_C2_Back>"
  Bus Selector1/94 -> BusCreator/313  "<IMAPve_g_L1_C1_Back>"
  Bus Selector1/93 -> BusCreator/312  "<IMAPve_g_L1_C0_Back>"
  Bus Selector1/92 -> BusCreator/311  "<IMAPve_g_R0_Range_FR_Pred>"
  Bus Selector1/91 -> BusCreator/310  "<IMAPve_g_R0_C2_FR_Pred>"
  Bus Selector1/90 -> BusCreator/309  "<IMAPve_g_R0_C1_FR_Pred>"
  Bus Selector1/89 -> BusCreator/308  "<IMAPve_g_R0_C0_FR_Pred>"
  Bus Selector1/88 -> BusCreator/307  "<IMAPve_g_R0_Range_Back>"
  Bus Selector1/87 -> BusCreator/306  "<IMAPve_g_R0_C3_Back>"
  Bus Selector1/86 -> BusCreator/305  "<IMAPve_g_R0_C2_Back>"
  Bus Selector1/85 -> BusCreator/304  "<IMAPve_g_R0_C1_Back>"
  Bus Selector1/84 -> BusCreator/303  "<IMAPve_g_R0_C0_Back>"
  Bus Selector1/83 -> BusCreator/302  "<IMAPve_g_L0_Range_FR_Pred>"
  Bus Selector1/82 -> BusCreator/301  "<IMAPve_g_L0_C2_FR_Pred>"
  Bus Selector1/81 -> BusCreator/300  "<IMAPve_g_L0_C1_FR_Pred>"
  Bus Selector1/80 -> BusCreator/299  "<IMAPve_g_L0_C0_FR_Pred>"
  Bus Selector1/79 -> BusCreator/298  "<IMAPve_g_L0_Range_Back>"
  Bus Selector1/78 -> BusCreator/297  "<IMAPve_g_L0_C3_Back>"
  Bus Selector1/77 -> BusCreator/296  "<IMAPve_g_L0_C2_Back>"
  Bus Selector1/76 -> BusCreator/295  "<IMAPve_g_L0_C1_Back>"
  Bus Selector1/75 -> BusCreator/294  "<IMAPve_g_L0_C0_Back>"
  Bus Selector1/74 -> BusCreator/293  "<IMAPve_d_R1_LC>"
  Bus Selector1/73 -> BusCreator/292  "<IMAPve_g_R1_TLC>"
  Bus Selector1/72 -> BusCreator/291  "<IMAPve_g_R1_W>"
  Bus Selector1/71 -> BusCreator/290  "<IMAPve_g_R1_Confidence>"
  Bus Selector1/70 -> BusCreator/289  "<IMAPve_d_R1_Type>"
  Bus Selector1/69 -> BusCreator/288  "<IMAPve_d_R1_Q>"
  Bus Selector1/68 -> BusCreator/287  "<IMAPve_g_R1_VR>"
  Bus Selector1/67 -> BusCreator/286  "<IMAPve_g_R1_C3>"
  Bus Selector1/66 -> BusCreator/285  "<IMAPve_g_R1_C2>"
  Bus Selector1/65 -> BusCreator/284  "<IMAPve_g_R1_C1>"
  Bus Selector1/64 -> BusCreator/283  "<IMAPve_g_R1_C0>"
  Bus Selector1/63 -> BusCreator/282  "<IMAPve_d_L1_LC>"
  Bus Selector1/62 -> BusCreator/281  "<IMAPve_g_L1_TLC>"
  Bus Selector1/61 -> BusCreator/280  "<IMAPve_g_L1_W>"
  Bus Selector1/60 -> BusCreator/279  "<IMAPve_g_L1_Confidence>"
  Bus Selector1/59 -> BusCreator/278  "<IMAPve_d_L1_Type>"
  Bus Selector1/58 -> BusCreator/277  "<IMAPve_d_L1_Q>"
  Bus Selector1/57 -> BusCreator/276  "<IMAPve_g_L1_VR>"
  Bus Selector1/56 -> BusCreator/275  "<IMAPve_g_L1_C3>"
  Bus Selector1/55 -> BusCreator/274  "<IMAPve_g_L1_C2>"
  Bus Selector1/54 -> BusCreator/273  "<IMAPve_g_L1_C1>"
  Bus Selector1/53 -> BusCreator/272  "<IMAPve_g_L1_C0>"
  Bus Selector1/52 -> BusCreator/271  "<IMAPve_d_R0_LC>"
  Bus Selector1/51 -> BusCreator/270  "<IMAPve_g_R0_TLC>"
  Bus Selector1/50 -> BusCreator/269  "<IMAPve_g_R0_W>"
  Bus Selector1/49 -> BusCreator/268  "<IMAPve_g_R0_Confidence>"
  Bus Selector1/48 -> BusCreator/267  "<IMAPve_d_R0_Type>"
  Bus Selector1/47 -> BusCreator/266  "<IMAPve_d_R0_Q>"
  Bus Selector1/46 -> BusCreator/265  "<IMAPve_g_R0_VR>"
  Bus Selector1/45 -> BusCreator/264  "<IMAPve_g_R0_C3>"
  Bus Selector1/44 -> BusCreator/263  "<IMAPve_g_R0_C2>"
  Bus Selector1/43 -> BusCreator/262  "<IMAPve_g_R0_C1>"
  Bus Selector1/42 -> BusCreator/261  "<IMAPve_g_R0_C0>"
  Bus Selector1/41 -> BusCreator/260  "<IMAPve_d_L0_LC>"
  Bus Selector1/40 -> BusCreator/259  "<IMAPve_g_L0_TLC>"
  Bus Selector1/39 -> BusCreator/258  "<IMAPve_g_L0_W>"
  Bus Selector1/38 -> BusCreator/257  "<IMAPve_g_L0_Confidence>"
  Bus Selector1/37 -> BusCreator/256  "<IMAPve_d_L0_Type>"
  Bus Selector1/36 -> BusCreator/255  "<IMAPve_d_L0_Q>"
  Bus Selector1/35 -> BusCreator/254  "<IMAPve_g_L0_VR>"
  Bus Selector1/34 -> BusCreator/253  "<IMAPve_g_L0_C3>"
  Bus Selector1/33 -> BusCreator/252  "<IMAPve_g_L0_C2>"
  Bus Selector1/32 -> BusCreator/251  "<IMAPve_g_L0_C1>"
  Bus Selector1/31 -> BusCreator/250  "<IMAPve_g_L0_C0>"
  Bus Selector1/30 -> BusCreator/249  "<IMAPve_d_ConsArea>"
  Bus Selector1/29 -> BusCreator/248  "<IMAPve_d_Road_Type>"
  Bus Selector1/28 -> BusCreator/247  "<IMAPve_d_Lane_Valid>"
  Bus Selector1/27 -> BusCreator/246  "<IMAPva_d_obj_MotionStatus>"
  Bus Selector1/26 -> BusCreator/245  "<IMAPva_d_obj_BrakeLight>"
  Bus Selector1/25 -> BusCreator/244  "<IMAPva_d_obj_TurnLight>"
  Bus Selector1/24 -> BusCreator/243  "<IMAPva_d_obj_age>"
  Bus Selector1/23 -> BusCreator/242  "<IMAPva_d_obj_status>"
  Bus Selector1/22 -> BusCreator/241  "<IMAPva_d_obj_lane>"
  Bus Selector1/21 -> BusCreator/240  "<IMAPva_d_obj_class>"
  Bus Selector1/20 -> BusCreator/239  "<IMAPva_g_obj_length>"
  Bus Selector1/19 -> BusCreator/238  "<IMAPva_g_obj_width>"
  Bus Selector1/18 -> BusCreator/237  "<IMAPva_g_obj_pos_var_xy>"
  Bus Selector1/17 -> BusCreator/236  "<IMAPva_g_obj_pos_var_y>"
  Bus Selector1/16 -> BusCreator/235  "<IMAPva_g_obj_pos_var_x>"
  Bus Selector1/15 -> BusCreator/234  "<IMAPva_g_obj_acc_y>"
  Bus Selector1/14 -> BusCreator/233  "<IMAPva_g_obj_acc_x>"
  Bus Selector1/13 -> BusCreator/232  "<IMAPva_g_obj_vel_y>"
  Bus Selector1/12 -> BusCreator/231  "<IMAPva_g_obj_vel_x>"
  Bus Selector1/11 -> BusCreator/230  "<IMAPva_g_obj_pos_y>"
  Bus Selector1/10 -> BusCreator/229  "<IMAPva_g_obj_pos_x>"
  Bus Selector1/9 -> BusCreator/228  "<IMAPva_d_obj_id>"
  Bus Selector1/8 -> BusCreator/227  "<IMAPve_d_obj_Num>"
  Bus Selector1/7 -> BusCreator/226  "<IMAPve_g_Fusion_Time_Stamp>"
  Bus Selector1/6 -> BusCreator/225  "<IMAPve_d_Fusion_Status>"
  Bus Selector1/5 -> BusCreator/224  "<IMAPve_d_RR_Radar_Status>"
  Bus Selector1/4 -> BusCreator/223  "<IMAPve_d_LR_Radar_Status>"
  Bus Selector1/3 -> BusCreator/222  "<IMAPve_d_RF_Radar_Status>"
  Bus Selector1/2 -> BusCreator/221  "<IMAPve_d_LF_Radar_Status>"
  Bus Selector1/1 -> BusCreator/220  "<IMAPve_d_Sensor_Status>"
  Ground4/1 -> BusCreator/158
  Ground3/1 -> BusCreator/157
  Ground2/1 -> BusCreator/156
  Ground1/1 -> BusCreator/155
  Bus Selector9/84 -> Terminator/1  "<IMAPve_g_FAPA_State>"
  Bus Selector9/79 -> BusCreator/145  "<IMAPve_d_Radar_State>"
  Bus Selector9/78 -> BusCreator/144  "<IMAPve_d_TPMS_Warn_Indicate>"
  Bus Selector9/77 -> BusCreator/143  "<IMAPve_d_TBOX_LocalTime_Valid>"
  Bus Selector9/76 -> BusCreator/142  "<IMAPve_d_TBOX_LocalTimeS>"
  Bus Selector9/75 -> BusCreator/141  "<IMAPve_d_TBOX_LocalTimeMin>"
  Bus Selector9/74 -> BusCreator/140  "<IMAPve_d_TBOX_LocalTimeH>"
  Bus Selector9/73 -> BusCreator/139  "<IMAPve_d_TBOX_LocalTimeD>"
  Bus Selector9/72 -> BusCreator/138  "<IMAPve_d_TBOX_LocalTimeM>"
  Bus Selector9/71 -> BusCreator/137  "<IMAPve_d_TBOX_LocalTimeY>"
  Bus Selector9/70 -> BusCreator/136  "<IMAPve_g_BCM_Battery_Voltage>"
  Bus Selector9/69 -> BusCreator/135  "<IMAPve_d_Radar_Detective_Req>"
  Bus Selector9/68 -> BusCreator/134  "<IMAPve_d_ESC_AVH_Status>"
  Bus Selector9/67 -> BusCreator/133  "<IMAPve_d_ESC_EBD_AlarmSig>"
  Bus Selector9/66 -> BusCreator/132  "<IMAPve_g_EPS_PowerCon>"
  Bus Selector9/65 -> BusCreator/131  "<IMAPve_d_EPS_Warning_State>"
  Bus Selector9/64 -> BusCreator/130  "<IMAPve_d_EPS_Steer_Hold_State>"
  Bus Selector9/63 -> BusCreator/129  "<IMAPve_d_ESC_Hold_State>"
  Bus Selector9/62 -> BusCreator/128  "<IMAPve_d_ESC_Drive_Direction>"
  Bus Selector9/61 -> BusCreator/127  "<IMAPve_d_EPB_Switch_Valid>"
  Bus Selector9/60 -> BusCreator/126  "<IMAPve_d_EPB_Switch_State>"
  Bus Selector9/59 -> BusCreator/125  "<IMAPve_d_EPB_Warn_Req>"
  Bus Selector9/58 -> BusCreator/124  "<IMAPve_d_EPB_Display_Req>"
  Bus Selector9/57 -> BusCreator/123  "<IMAPve_d_EPB_Status>"
  Bus Selector9/56 -> BusCreator/122  "<IMAPve_d_BCM_HighBeam_State>"
  Bus Selector9/55 -> BusCreator/121  "<IMAPve_d_BCM_LowBeam_State>"
  Bus Selector9/54 -> BusCreator/120  "<IMAPve_d_EMS_Brake_Pedal>"
  Bus Selector9/53 -> BusCreator/119  "<IMAPve_d_EMS_ACC_Inhibited>"
  Bus Selector9/52 -> BusCreator/118  "<IMAPve_d_EMS_ACC_CtlAvail>"
  Bus Selector9/51 -> BusCreator/117  "<IMAPve_d_ACU_Passenger_Belt>"
  Bus Selector9/50 -> BusCreator/116  "<IMAPve_d_GW_Brake_Only_Req>"
  Bus Selector9/49 -> BusCreator/115  "<IMAPve_d_BCM_BrakeLamp_State>"
  Bus Selector9/48 -> BusCreator/114  "<IMAPve_d_BCM_CHMSL_Status>"
  Bus Selector9/47 -> BusCreator/113  "<IMAPve_d_BCM_FrontWiper_State>"
  Bus Selector9/46 -> BusCreator/112  "<IMAPve_d_EMS_ACC_Effective>"
  Bus Selector9/45 -> BusCreator/111  "<IMAPve_d_ESC_ACC_Active>"
  Bus Selector9/44 -> BusCreator/110  "<IMAPve_d_ESC_ACC_Available>"
  Bus Selector9/43 -> BusCreator/109  "<IMAPve_d_ESC_ACC_Status>"
  Bus Selector9/42 -> BusCreator/108  "<IMAPve_d_ESC_AEB_Active>"
  Bus Selector9/41 -> BusCreator/107  "<IMAPve_d_ESC_AEB_Available>"
  Bus Selector9/40 -> BusCreator/106  "<IMAPve_d_ESC_AEB_Status>"
  Bus Selector9/39 -> BusCreator/105  "<IMAPve_d_ESC_Brake_Failsafe>"
  Bus Selector9/38 -> BusCreator/104  "<IMAPve_d_EMS_Gearbox_CtlAvail>"
  Bus Selector9/37 -> BusCreator/103  "<IMAPve_d_EMS_Engine_Status>"
  Bus Selector9/36 -> BusCreator/102  "<IMAPve_d_TCU_Select_ATMode>"
  Bus Selector9/35 -> BusCreator/101  "<IMAPve_d_TCU_Gear_Engage>"
  Bus Selector9/34 -> BusCreator/100  "<IMAPve_d_TCU_DCT_Clutch_State>"
  Bus Selector9/33 -> BusCreator/99  "<IMAPve_d_TCU_Shift_Valid>"
  Bus Selector9/32 -> BusCreator/98  "<IMAPve_d_TCU_AT_Failure>"
  Bus Selector9/31 -> BusCreator/97  "<IMAPve_d_ESC_RR_Wheel_Pulse>"
  Bus Selector9/30 -> BusCreator/96  "<IMAPve_d_ESC_RL_Wheel_Pulse>"
  Bus Selector9/29 -> BusCreator/95  "<IMAPve_d_ESC_FR_Wheel_Pulse>"
  Bus Selector9/28 -> BusCreator/94  "<IMAPve_d_ESC_FL_Wheel_Pulse>"
  Bus Selector9/27 -> BusCreator/93  "<IMAPve_d_ESC_RR_WhlSpd_Fault>"
  Bus Selector9/26 -> BusCreator/92  "<IMAPve_g_ESC_RR_WhlSpd>"
  Bus Selector9/25 -> BusCreator/91  "<IMAPve_d_ESC_RL_WhlSpd_Fault>"
  Bus Selector9/24 -> BusCreator/90  "<IMAPve_g_ESC_RL_WhlSpd>"
  Bus Selector9/23 -> BusCreator/89  "<IMAPve_d_ESC_FR_WhlSpd_Fault>"
  Bus Selector9/22 -> BusCreator/88  "<IMAPve_g_ESC_FR_WhlSpd>"
  Bus Selector9/21 -> BusCreator/87  "<IMAPve_d_ESC_FL_WhlSpd_Fault>"
  Bus Selector9/20 -> BusCreator/86  "<IMAPve_g_ESC_FL_WhlSpd>"
  Bus Selector9/19 -> BusCreator/85  "<IMAPve_d_ESC_RR_WheelPulVal>"
  Bus Selector9/18 -> BusCreator/84  "<IMAPve_d_ESC_RL_WheelPulVal>"
  Bus Selector9/17 -> BusCreator/83  "<IMAPve_d_ESC_FR_WheelPulVal>"
  Bus Selector9/16 -> BusCreator/82  "<IMAPve_d_ESC_FL_WheelPulVal>"
  Bus Selector9/15 -> BusCreator/81  "<IMAPve_d_ESC_ABS_AlarmSig>"
  Bus Selector9/14 -> BusCreator/80  "<IMAPve_d_ESC_ABS_Valid>"
  Bus Selector9/13 -> BusCreator/79  "<IMAPve_d_ESC_ABS_Active>"
  Bus Selector9/12 -> BusCreator/78  "<IMAPve_d_Brake_Pedal_Fault>"
  Bus Selector9/11 -> BusCreator/77  "<IMAPve_d_ESC_VehSpd_Valid>"
  Bus Selector9/10 -> BusCreator/76  "<IMAPve_d_ESC_TCS_Active>"
  Bus Selector9/9 -> BusCreator/75  "<IMAPve_d_ESC_MSR_Active>"
  Bus Selector9/8 -> BusCreator/74  "<IMAPve_d_ESC_ESC_Active>"
  Bus Selector9/7 -> BusCreator/73  "<IMAPve_d_Speed_Limit_Switch>"
  Bus Selector9/6 -> BusCreator/72  "<IMAPve_d_ESC_AlarmSig>"
  Bus Selector9/5 -> BusCreator/71  "<IMAPve_d_ESC_OFF>"
  Bus Selector9/4 -> BusCreator/70  "<IMAPve_d_SWS_Failure_Status>"
  Bus Selector9/3 -> BusCreator/69  "<IMAPve_d_SWS_Fault_Code>"
  Bus Selector9/2 -> BusCreator/68  "<IMAPve_d_ACU_Driver_Belt>"
  Bus Selector9/1 -> BusCreator/67  "<IMAPve_d_BCM_Ignition_State>"
  Bus Selector9/80 -> BusCreator/146  "<IMAPve_d_ACC_Desired_Headway>"
  Bus Selector9/81 -> BusCreator/147  "<IMAPve_d_Time_System_Clock>"
  Bus Selector9/82 -> BusCreator/148  "<IMAPve_d_Signal_Time_Stamp>"
  Bus Selector9/83 -> BusCreator/150  "<IMAPve_g_GW_IC_Odometer>"
  Bus Selector9/85 -> BusCreator/151  "<IMAPve_d_Outside_Temp>"
  [FDMMve_d_AccFcnConf] -> BusCreator/153
  [ICABva_d_ICAB2ACCS] -> BusCreator/154
  [ICAS_output] -> Bus Selector2/1
  Bus Selector11/40 -> BusCreator/216  "<IMAPve_g_ORI_R1_VR>"
  Bus Selector11/39 -> BusCreator/215  "<IMAPve_d_ORI_R1_LT>"
  Bus Selector11/43 -> BusCreator/219  "<IMAPve_d_ORI_R1_LC>"
  Bus Selector11/42 -> BusCreator/218  "<IMAPve_g_ORI_R1_W>"
  Bus Selector11/41 -> BusCreator/217  "<IMAPve_g_ORI_R1_TLC>"
  Bus Selector11/38 -> BusCreator/214  "<IMAPve_d_ORI_R1_Q>"
  Bus Selector11/37 -> BusCreator/213  "<IMAPve_g_ORI_R1_C0>"
  Bus Selector11/36 -> BusCreator/212  "<IMAPve_g_ORI_R1_C1>"
  Bus Selector11/35 -> BusCreator/211  "<IMAPve_g_ORI_R1_C2>"
  Bus Selector11/34 -> BusCreator/210  "<IMAPve_g_ORI_R1_C3>"
  Bus Selector11/33 -> BusCreator/209  "<IMAPve_d_ORI_R0_LC>"
  Bus Selector11/32 -> BusCreator/208  "<IMAPve_g_ORI_R0_W>"
  Bus Selector11/31 -> BusCreator/207  "<IMAPve_g_ORI_R0_TLC>"
  Bus Selector11/30 -> BusCreator/206  "<IMAPve_g_ORI_R0_VR>"
  Bus Selector11/29 -> BusCreator/205  "<IMAPve_d_ORI_R0_LT>"
  Bus Selector11/28 -> BusCreator/204  "<IMAPve_d_ORI_R0_Q>"
  Bus Selector11/27 -> BusCreator/203  "<IMAPve_g_ORI_R0_C0>"
  Bus Selector11/26 -> BusCreator/202  "<IMAPve_g_ORI_R0_C1>"
  Bus Selector11/25 -> BusCreator/201  "<IMAPve_g_ORI_R0_C2>"
  Bus Selector11/24 -> BusCreator/200  "<IMAPve_g_ORI_R0_C3>"
  Bus Selector11/23 -> BusCreator/199  "<IMAPve_d_ORI_L1_LC>"
  Bus Selector11/22 -> BusCreator/198  "<IMAPve_g_ORI_L1_W>"
  Bus Selector11/21 -> BusCreator/197  "<IMAPve_g_ORI_L1_TLC>"
  Bus Selector11/20 -> BusCreator/196  "<IMAPve_g_ORI_L1_VR>"
  Bus Selector11/19 -> BusCreator/195  "<IMAPve_d_ORI_L1_Type>"
  Bus Selector11/18 -> BusCreator/194  "<IMAPve_d_ORI_L1_Q>"
  Bus Selector11/17 -> BusCreator/193  "<IMAPve_g_ORI_L1_C0>"
  Bus Selector11/16 -> BusCreator/192  "<IMAPve_g_ORI_L1_C1>"
  Bus Selector11/15 -> BusCreator/191  "<IMAPve_g_ORI_L1_C2>"
  Bus Selector11/14 -> BusCreator/190  "<IMAPve_g_ORI_L1_C3>"
  Bus Selector11/13 -> BusCreator/189  "<IMAPve_d_ORI_L0_LC>"
  Bus Selector11/12 -> BusCreator/188  "<IMAPve_g_ORI_L0_W>"
  Bus Selector11/11 -> BusCreator/187  "<IMAPve_g_ORI_L0_TLC>"
  Bus Selector11/10 -> BusCreator/186  "<IMAPve_g_ORI_L0_VR>"
  Bus Selector11/9 -> BusCreator/185  "<IMAPve_d_ORI_L0_Type>"
  Bus Selector11/8 -> BusCreator/184  "<IMAPve_d_ORI_L0_Q>"
  Bus Selector11/7 -> BusCreator/183  "<IMAPve_g_ORI_L0_C0>"
  Bus Selector11/6 -> BusCreator/182  "<IMAPve_g_ORI_L0_C1>"
  Bus Selector11/5 -> BusCreator/181  "<IMAPve_g_ORI_L0_C2>"
  Bus Selector11/4 -> BusCreator/180  "<IMAPve_g_ORI_L0_C3>"
  Bus Selector11/3 -> BusCreator/179  "<IMAPve_d_ORI_Lane_RoadType>"
  Bus Selector11/2 -> BusCreator/178  "<IMAPve_d_ORI_Lane_ConsArea>"
  Bus Selector11/1 -> BusCreator/177  "<IMAPve_d_ORI_Lane_Valid>"
  [IMAP_ORI_Lane] -> Bus Selector11/1
  Bus Selector10/12 -> BusCreator/176  "<IMAPva_d_ORI_Obj_ID>"
  Bus Selector10/11 -> BusCreator/175  "<IMAPva_g_ORI_Obj_Width>"
  Bus Selector10/10 -> BusCreator/174  "<IMAPva_g_ORI_Obj_RAngle>"
  Bus Selector10/9 -> BusCreator/173  "<IMAPva_g_ORI_Obj_LAngle>"
  Bus Selector10/8 -> BusCreator/172  "<IMAPva_d_ORI_Obj_Lane>"
  Bus Selector10/7 -> BusCreator/171  "<IMAPva_g_ORI_Obj_LongDis>"
  Bus Selector10/6 -> BusCreator/170  "<IMAPva_g_ORI_Obj_RelVel>"
  Bus Selector10/5 -> BusCreator/169  "<IMAPva_d_ORI_Obj_Motion>"
  Bus Selector10/4 -> BusCreator/168  "<IMAPva_d_ORI_Obj_Class>"
  Bus Selector10/3 -> BusCreator/167  "<IMAPva_g_ORI_Probability>"
  Bus Selector10/2 -> BusCreator/166  "<IMAPve_d_ORI_Obj_Num>"
  Bus Selector10/1 -> BusCreator/165  "<IMAPve_d_ORI_CIPV_ID>"
  [IMAP_ORI_obj] -> Bus Selector10/1
  Clock/1 -> Data Type Conversion/1  "TIME_System_Clock"
  [IMAP_State] -> Bus Selector9/1
  Bus Selector8/20 -> BusCreator/66  "<IMAPve_d_TCU_PRND_State>"
  Bus Selector8/19 -> BusCreator/65  "<IMAPve_d_TCU_Target_Gear>"
  Bus Selector8/18 -> BusCreator/64  "<IMAPve_d_TCU_Actual_Gear>"
  Bus Selector8/17 -> BusCreator/63  "<IMAPve_d_ESC_Veh_Standstill>"
  Bus Selector8/16 -> BusCreator/62  "<IMAPve_g_EMS_Engine_Speed>"
  Bus Selector8/15 -> BusCreator/61  "<IMAPve_d_ESC_Brake_Effort>"
  Bus Selector8/14 -> BusCreator/60  "<IMAPve_g_EMS_Driver_Torque>"
  Bus Selector8/13 -> BusCreator/59  "<IMAPve_d_EMS_AccPedal_Fault>"
  Bus Selector8/12 -> BusCreator/58  "<IMAPve_g_EMS_ACC_VirtualPedal>"
  Bus Selector8/11 -> BusCreator/57  "<IMAPve_g_EMS_Realize_TWhl>"
  Bus Selector8/10 -> BusCreator/56  "<IMAPve_g_EMS_Actual_IndT>"
  Bus Selector8/9 -> BusCreator/55  "<IMAPve_g_EMS_Actual_FlwT>"
  Bus Selector8/8 -> BusCreator/54  "<IMAPve_g_EMS_MinTWhl_Offset>"
  Bus Selector8/7 -> BusCreator/53  "<IMAPve_g_EMS_MinTWhl>"
  Bus Selector8/6 -> BusCreator/52  "<IMAPve_g_EMS_MaxTWhl_Offset>"
  Bus Selector8/5 -> BusCreator/51  "<IMAPve_g_EMS_MaxTWhl>"
  Bus Selector8/4 -> BusCreator/50  "<IMAPve_g_EMS_RealPedal>"
  Bus Selector8/3 -> BusCreator/49  "<IMAPve_g_EMS_Pot_WhlT_Min>"
  Bus Selector8/2 -> BusCreator/48  "<IMAPve_g_EMS_Pot_WhlT_Max>"
  Bus Selector8/1 -> BusCreator/47  "<IMAPve_d_EMS_ACC_Status>"
  [IMAP_bsPTState] -> Bus Selector8/1
  Bus Selector7/4 -> BusCreator/46  "<IMAPve_d_BCM_Door_Lock_State>"
  Bus Selector7/3 -> BusCreator/45  "<IMAPve_d_PEPS_Door_Lock_Req>"
  Bus Selector7/2 -> BusCreator/44  "<IMAPve_d_SCC_Right_SwitchSig>"
  Bus Selector7/1 -> BusCreator/43  "<IMAPve_d_SCC_Left_SwitchSig>"
  [IMAP_FKeyStRx] -> Bus Selector7/1
  Bus Selector6/10 -> BusCreator/42  "<IMAPve_d_BCM_LR_Door_State>"
  Bus Selector6/9 -> BusCreator/41  "<IMAPve_d_BCM_RR_Door_State>"
  Bus Selector6/8 -> BusCreator/40  "<IMAPve_d_BCM_RF_Door_State>"
  Bus Selector6/7 -> BusCreator/39  "<IMAPve_d_BCM_LF_Door_State>"
  Bus Selector6/6 -> BusCreator/38  "<IMAPve_d_BCM_Trunk_State>"
  Bus Selector6/5 -> BusCreator/37  "<IMAPve_d_BCM_Opening_State>"
  Bus Selector6/4 -> BusCreator/36  "<IMAPve_d_ESC_BrakeLamp_Req>"
  Bus Selector6/3 -> BusCreator/35  "<IMAPve_d_BCM_Right_Light>"
  Bus Selector6/2 -> BusCreator/34  "<IMAPve_d_BCM_Left_Light>"
  Bus Selector6/1 -> BusCreator/33  "<IMAPve_d_BCM_HazardLamp>"
  [IMAP_BESRx] -> Bus Selector6/1
  Bus Selector5/1 -> BusCreator/31  "<IMAPve_g_SW_Angle>"
  Bus Selector5/2 -> BusCreator/32  "<IMAPve_g_SW_Angle_Speed>"
  [IMAP_SWARx] -> Bus Selector5/1
  Bus Selector4/12 -> BusCreator/30  "<IMAPve_g_ESC_DySlope>"
  Bus Selector4/11 -> BusCreator/29  "<IMAPve_g_ESC_DySlope_Accuracy>"
  Bus Selector4/10 -> BusCreator/28  "<IMAPve_g_ESC_Static_Slope>"
  Bus Selector4/9 -> BusCreator/27  "<IMAPve_g_ESC_Brake_Press>"
  Bus Selector4/8 -> BusCreator/26  "<IMAPve_d_ESC_LonAcc_Valid>"
  Bus Selector4/7 -> BusCreator/25  "<IMAPve_g_ESC_LonAcc>"
  Bus Selector4/6 -> BusCreator/24  "<IMAPve_g_ESC_VehSpd>"
  Bus Selector4/5 -> BusCreator/23  "<IMAPve_g_ESC_UnYawRate>"
  Bus Selector4/4 -> BusCreator/22  "<IMAPve_d_ESC_YawRate_Valid>"
  Bus Selector4/3 -> BusCreator/21  "<IMAPve_g_ESC_YawRate>"
  Bus Selector4/2 -> BusCreator/20  "<IMAPve_d_ESC_LatAcc_Valid>"
  Bus Selector4/1 -> BusCreator/19  "<IMAPve_g_ESC_LatAcc>"
  [IMAP_VehMovRx] -> Bus Selector4/1
  Bus Selector3/8 -> BusCreator/18  "<IMAPve_g_EPS_LKA_Current>"
  Bus Selector3/7 -> BusCreator/17  "<IMAPve_d_EPS_TrqLim_State>"
  Bus Selector3/6 -> BusCreator/16  "<IMAPve_d_SAS_Trim_State>"
  Bus Selector3/5 -> BusCreator/15  "<IMAPve_d_SAS_Clb_State>"
  Bus Selector3/4 -> BusCreator/14  "<IMAPve_d_EPS_Trq_State>"
  Bus Selector3/3 -> BusCreator/13  "<IMAPve_d_EPS_Error_State>"
  Bus Selector3/2 -> BusCreator/12  "<IMAPve_g_EPS_SW_Trq>"
  Bus Selector3/1 -> BusCreator/11  "<IMAPve_d_EPS_LKA_State>"
  [IMAP_EPSRx] -> Bus Selector3/1
  Bus Selector/10 -> BusCreator/10  "<IMAPve_d_ALC_Sensitivity>"
  Bus Selector/9 -> BusCreator/9  "<IMAPve_d_ICA_Config>"
  Bus Selector/8 -> BusCreator/8  "<IMAPve_d_LF_Switch>"
  Bus Selector/7 -> BusCreator/7  "<IMAPve_d_DOW_Switch>"
  Bus Selector/6 -> BusCreator/6  "<IMAPve_d_PEPS_RKE_Command>"
  Bus Selector/5 -> BusCreator/5  "<IMAPve_d_ALC_TLC_Mode>"
  Bus Selector/4 -> BusCreator/4  "<IMAPve_d_Speed_Limit>"
  Bus Selector/3 -> BusCreator/3  "<IMAPve_d_ISA_ISLC_Mode>"
  Bus Selector/2 -> BusCreator/2  "<IMAPve_d_TSR_Switch>"
  Bus Selector/1 -> BusCreator/1  "<IMAPve_d_ISA_Switch>"
  [IMAP_MP5Rx] -> Bus Selector/1
  [IMAP_Fusion_Sig] -> Bus Selector1/1
  BusCreator/1 -> To Workspace/1
